simulink model "RcModel"  (R2020a)
settings: Solver=FixedStepAuto  StartTime=0.0  StopTime=3  FixedStep=0.001  MaxStep=1e-3  RelTol=1e-3  AbsTol=1e-3
PreLoadFcn:
  | R=1000;
  | C=100e-6;
CloseFcn:
  | try,close(h1_ssc_rc_circuit_sl),end
  | clear h1_ssc_rc_circuit_sl
  | clear simlog_ssc_rc_circuit_sl
  | clear logsout_ssc_rc_circuit_sl
Description:
  | RC Circuit model derived by Mathworks model
  | 
  | https://it.mathworks.com/help/physmod/simscape/examples/rc-circuit-in-simulink-and-simscape.html
settings Model: ModifiedHistory=First implementation  Creator=AA  LastModifiedBy=ubuntu
settings SolverCC: AutoScaleAbsTol=off  NumberNewtonIterations=2  SolverJacobianMethodControl=FullAnalytical
settings DataIOCC: LimitDataPoints=on  SaveFormat=Array  ReturnWorkspaceOutputs=off  SignalLoggingName=logsout_ssc_rc_circuit_sl
settings DebuggingCC: SolverPrmCheckMsg=warning  AllowSymbolicDim=off  PregeneratedLibrarySubsystemCodeDiagnostic=none  SFUnexpectedBacktrackingDiag=warning  SFNoUnconditionalDefaultTransitionDiag=warning  SFExecutionAtInitializationDiag=none  ArithmeticOperatorsInVariantConditions=warning
settings HardwareCC: ProdBitPerPointer=32  ProdBitPerSizeT=32  ProdBitPerPtrDiffT=32  ProdLargestAtomicFloat=None  ProdIntDivRoundTo=Undefined  ProdEndianess=Unspecified  ProdWordSize=32  ProdHWDeviceType=32-bit Generic
settings ModelReferenceCC: PropagateSignalLabelsOutOfModel=off
settings SFSimCC: SimUseLocalCustomCode=off  CustomCodeUndefinedFunction=UseInterfaceOnly
settings RTWCC: Description=Generic Real-Time Target  RTWUseLocalCustomCode=off
settings CodeAppCC: StateflowObjectComments=on
settings GRTTargetCC: TargetLangStandard=C89/C90 (ANSI)
settings ConfigComp: CovMetricSettings=dw  CovHtmlReporting=on  CovSaveCumulativeToWorkspaceVar=on  CovSaveSingleToWorkspaceVar=on  CovExternalEMLEnable=off  CovSFcnEnable=off
settings SimscapeCC: SimscapeLogType=all  SimscapeLogSimulationStatistics=on  SimscapeLogName=simlog_ssc_rc_circuit_sl  SimscapeLogLimitData=off  SimscapeLogDataHistory=10000

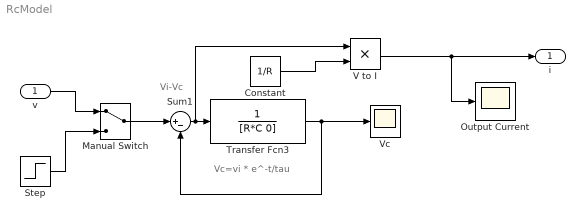
== system RcModel ==
  note: Vi-Vc
  note: Vc=vi * e^-t/tau
  v : Inport
  Constant : Constant  Value=1/R
  Manual Switch : ManualSwitch
  Output Current : Scope
  Step : Step  SampleTime=0
  Sum1 : Sum  Inputs=|+-
  Transfer Fcn3 : TransferFcn  InitFcn=wp=1/(R*C);  Denominator=[R*C 0]
  V to I : Product  InputSameDT=on
  Vc : Scope
  i : Outport
  wires:
  Sum1/1 -> V to I/1, Transfer Fcn3/1
  Transfer Fcn3/1 -> Sum1/2, Vc/1
  V to I/1 -> i/1, Output Current/1
  Constant/1 -> V to I/2
  v/1 -> Manual Switch/1
  Manual Switch/1 -> Sum1/1
  Step/1 -> Manual Switch/2
